simulink model "pumaModel"  (R2021b)
settings: Solver=VariableStepAuto  StartTime=0.0  StopTime=stopTime  FixedStep=.0001  RelTol=1e-3
values from neighbouring files (symbols this model uses):
  C = [0 c12_1*dq1 c13_1*dq3;c11_2*dq1 0 c22_2*dq2+c23_2*dq3;c11_3*dq1 c22_3*dq2 0]    [puma560ModifiedDynamics.m]
  dq_0 = [0 0 0]    [matlab.mat]
  fdControl = 2    [InitializationScript.m]
  fEE = 0    [InitializationScript.m]    (also in matlab.mat = 100)
  IC = [0;0;0]    [InitializationScript.m]    (also in matlab.mat = [0 0 0])
  m = 3    [matlab.mat]
  pathPoints = [IC,solution1,solution2,solution3,solution4,solution5,solution6]    [InitializationScript.m]    (also in matlab.mat = [0 0 0 4.71238898038 -1.57079632679 3.14159265359 3.14159265)
  q_0 = [0 0 0]    [matlab.mat]
  timePoints = [0 2 4 6 8 10 12]    [InitializationScript.m]    (also in matlab.mat = [0 2 4 6 8])
  velPoints = zeros(3,7)    [InitializationScript.m]    (also in matlab.mat = [0 0 0 0 0 0 0 0 0 0 0 0 ... (15 elements, 3x5)])
  X = [cos(q1)*(l2*cos(q2)+l3*sin(q2+q3));sin(q1)*(l2*cos(q2)+l3*sin(q2+q3));l1-l2*sin(q2)+l3*cos(q2+q3)]    [puma560ModifiedDynamics.m]
  Y = sym(zeros(3,size(cat(2,Y1,Y2,Y3),2)))    [puma560ModifiedDynamics.m]
undefined symbols (not defined in the file or in its folder): Z
libraries: sm_lib x96, nesl_utility x60, simulink x7, robotmaniplib x1, robotcorelib x1
(part 1 of 5)
PostSaveFcn:
  | save VariantSettings.mat
settings Model: VariantConfigurationObject=PUMA560VariantSettings  Creator=Chris  LastModifiedBy=Chris
settings SolverCC: AlgebraicLoopSolver=LineSearch
settings DebuggingCC: SFMachineParentedDataDiag=warning

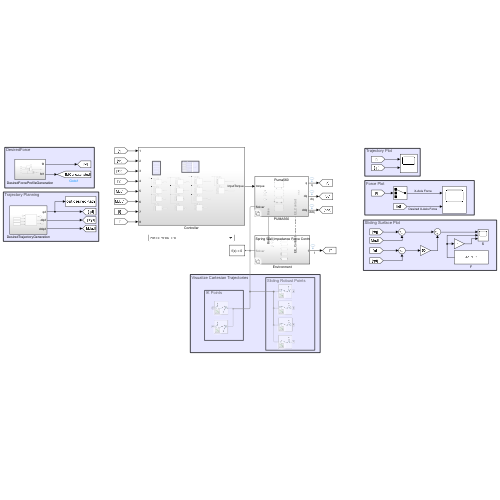
[thumbnail: Simulink's stored preview of the top-level diagram]
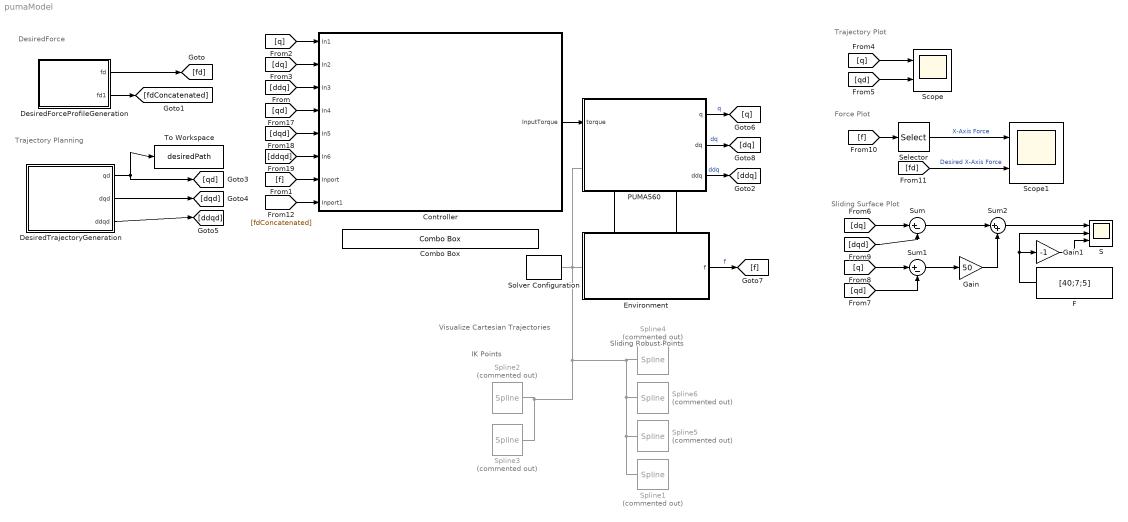
== system pumaModel ==
  note: Visualize Cartesian Trajectories
  note: DesiredForce
  note: Sliding Surface Plot
  note: Trajectory Plot
  note: Sliding Robust Points
  note: IK Points
  note: Trajectory Planning
  note: Force Plot
  Combo Box : ComboBox  LabelPosition=Hide  SelectedLabel=Parrellel Motion Force
      settings: Values={{'Inverse Torque', 'Lyapunov Torque', 'Impedance Joint Space', 'Impedance Task Space', 'Adaptive Control', 'PD + Gravity', 'Impedance Task State', 'Robust Control', 'Parrellel Motion Force', 'Task Space Impedance With Measurements', 'Sliding Robust Controller', 'Hybrid Force Motion', 'Hybrid Impedance Motion Control', 'Hybrid Impedance Force Control'}, [1 2 3 4 5 6 7 8 9 10 11 12 13 14]}
  Controller : Subsystem
  DesiredForceProfileGeneration : Subsystem
  DesiredTrajectoryGeneration : Subsystem
  Environment : Subsystem  Variant=on
      settings: PortSchema="{\"entries\":[{\"content\":{\"sides\":[{\"content\":{\"connectorIds\":[\"LConn1\"]},\"type\":\"ConnectorPlacement.EquallySpacedRectSide\",\"uuid\":\"bb63e962-d15f-4f0f-af2b-d9166a575433\"},{\"content\":{\"connectorIds\":[\"Out1\"],\"side\":\"RIGHT\"},\"type\":\"ConnectorPlacement.EquallySpacedRectSide\",\"uuid\":\"5f217ea6-af7d-4c7c-9fae-005e6a80c75a\"},{\"content\":{\"connectorIds\":[\"LConn2\",\"LConn3\"],\"side\":\"TOP\"},\"type\":\"ConnectorPlacement.EquallySpacedRectSide\",\"uuid\":\"72e5d329-ee37-4049-b27a-f006421b2cb1\"},{\"content\":{\"connectorIds\":[],\"side\":\"HIDDEN\"},\"type\":\"ConnectorPlacement.EquallySpacedRectSide\",\"uuid\":\"fb212f45-e29a-441e-a219-fbabe0f84998\"}]},\"type\":\"ConnectorPlacement.EquallySpacedConnector\",\"uuid\":\"6d8f9ed1-4648-49c1-a401-abad2abde741\"}],\"packageUris\":[\"http://schema.mathworks.com/mf0/Connector/R2020b\"],\"version\":\"1.0\"}"
  F : Constant  Value=[40;7;5]
  Gain : Gain  Gain=50
  Gain1 : Gain  Gain=-1
  PUMA560 : Subsystem  Variant=on
      settings: PortSchema="{\"entries\":[{\"content\":{\"sides\":[{\"content\":{\"connectorIds\":[\"In1\",\"LConn1\"]},\"type\":\"ConnectorPlacement.EquallySpacedRectSide\",\"uuid\":\"c7b40478-8afa-4d90-abdc-2a1179e0c85a\"},{\"content\":{\"connectorIds\":[\"Out1\",\"Out2\",\"Out3\"],\"side\":\"RIGHT\"},\"type\":\"ConnectorPlacement.EquallySpacedRectSide\",\"uuid\":\"fe05b273-9859-45af-b8f0-bcdecff42ea9\"},{\"content\":{\"connectorIds\":[],\"side\":\"TOP\"},\"type\":\"ConnectorPlacement.EquallySpacedRectSide\",\"uuid\":\"8295939b-ed6c-494a-8f2d-0843651cca51\"},{\"content\":{\"connectorIds\":[\"RConn1\",\"RConn2\"],\"side\":\"BOTTOM\"},\"type\":\"ConnectorPlacement.EquallySpacedRectSide\",\"uuid\":\"fbe51ea0-cfb2-4db3-ab8e-748ba1c11ce6\"},{\"content\":{\"connectorIds\":[],\"side\":\"HIDDEN\"},\"type\":\"ConnectorPlacement.EquallySpacedRectSide\",\"uuid\":\"fa6272a3-c07c-42c1-8bc0-64c7f45ab8c0\"}]},\"type\":\"ConnectorPlacement.EquallySpacedConnector\",\"uuid\":\"730599d1-a108-4fea-aae7-88428ae8f259\"}],\"packageUris\":[\"http://schema.mathworks.com/mf0/Connector/R2020b\"],\"version\":\"1.0\"}"
  S : Scope  NumInputPorts=3
  Scope : Scope  NumInputPorts=2
  Scope1 : Scope  NumInputPorts=2
  Selector : Selector  InputPortWidth=3  IndexOptions=Index vector (dialog)  Indices=[1]  OutputSizes=1
  Solver Configuration : nesl_utility/Solver Configuration  PhysicalDomain=network_engine_domain  SubClassName=solver  LeftPortType=input  RightPortType=generic  Tones=[]  Harmonics=[]  SimulateNoise=off  Profile=off  UseLocalSampling=off  EnableSwitchedLinearOptims=on  FrequencyDomain=off  UseCCode=off  RelTol=0.001  AbsTol=1e-06  MinStep=1e-09  ToWorkspace=off  RevertToSquareIcSolve=off  NumHomotopyIterations=100  PhasorMode=off  PhasorModeNumHarmonics=1  DoDC=off  ResidualTolerance=1e-09  UseLocalSolver=off  LocalSolverChoice=NE_PARTITIONING_ADVANCER  LocalSolverSampleTime=0.001  DoFixedCost=off  MaxNonlinIter=3  MaxModeIter=2  ComputeImpulses=off  ImpulseIterations=2  LinearAlgebra=auto  EquationFormulation=NE_TIME_EF  DelaysMemoryBudget=1024  AutomaticFiltering=on  FilteringTimeConstant=0.001  PartitionStorageMethod=AS_NEEDED  PartitionMemoryBudget=1024  PartitionMethod=ROBUST
      settings: SourceProductBaseCode=PW,SS
  Spline1 : sm_lib/Curves and Surfaces/Spline  Commented=on  GraphicAmbientColor=[0.15 0.15 0.15 1.0]  GraphicDiffuseColor=[1.0 1.0 0.0]  DataPoints=out.xTrajectory.Data  DataPointsUnits=m  GraphicEmissiveColor=[0.0 0.0 0.0 1.0]  EndConditionType=Natural  MarkerShape=Sphere  MarkerSize=10  GraphicType=FromGeometry  GraphicOpacity=1.0  GraphicShininess=75  GraphicSpecularColor=[0.5 0.5 0.5 1.0]  GraphicVisPropType=SimpleVisualProperties
  Spline2 : sm_lib/Curves and Surfaces/Spline  Commented=on  GraphicAmbientColor=[0.15 0.15 0.15 1.0]  GraphicDiffuseColor=[0.2 1.0 0.0]  DataPoints=preSetPointsDesired  DataPointsUnits=m  GraphicEmissiveColor=[0.0 0.0 0.0 1.0]  EndConditionType=Natural  MarkerShape=Sphere  MarkerSize=10  GraphicType=FromGeometry  GraphicOpacity=1.0  GraphicShininess=75  GraphicSpecularColor=[0.5 0.5 0.5 1.0]  GraphicVisPropType=SimpleVisualProperties
  Spline3 : sm_lib/Curves and Surfaces/Spline  Commented=on  GraphicAmbientColor=[0.15 0.15 0.15 1.0]  GraphicDiffuseColor=[1.0 0.0 0.2]  DataPoints=preSetPointsIK  DataPointsUnits=m  GraphicEmissiveColor=[0.0 0.0 0.0 1.0]  EndConditionType=Natural  MarkerShape=Sphere  MarkerSize=10  GraphicType=FromGeometry  GraphicOpacity=1.0  GraphicShininess=75  GraphicSpecularColor=[0.5 0.5 0.5 1.0]  GraphicVisPropType=SimpleVisualProperties
  Spline4 : sm_lib/Curves and Surfaces/Spline  Commented=on  GraphicAmbientColor=[0.15 0.15 0.15 1.0]  GraphicDiffuseColor=[1.0 0.0 0.2]  DataPoints=robustControlPoints_IK  DataPointsUnits=m  GraphicEmissiveColor=[0.0 0.0 0.0 1.0]  EndConditionType=Natural  MarkerShape=Sphere  MarkerSize=10  GraphicType=FromGeometry  GraphicOpacity=1.0  GraphicShininess=75  GraphicSpecularColor=[0.5 0.5 0.5 1.0]  GraphicVisPropType=SimpleVisualProperties
  Spline5 : sm_lib/Curves and Surfaces/Spline  Commented=on  GraphicAmbientColor=[0.15 0.15 0.15 1.0]  GraphicDiffuseColor=[0.0 1.0 0.2]  DataPoints=fEEPoints  DataPointsUnits=m  GraphicEmissiveColor=[0.0 0.0 0.0 1.0]  EndConditionType=Natural  MarkerShape=Sphere  MarkerSize=10  GraphicType=FromGeometry  GraphicOpacity=1.0  GraphicShininess=75  GraphicSpecularColor=[0.5 0.5 0.5 1.0]  GraphicVisPropType=SimpleVisualProperties
  Spline6 : sm_lib/Curves and Surfaces/Spline  Commented=on  GraphicAmbientColor=[0.15 0.15 0.15 1.0]  GraphicDiffuseColor=[1.0 1.0 0.0]  DataPoints=robustControlPoints  DataPointsUnits=m  GraphicEmissiveColor=[0.0 0.0 0.0 1.0]  EndConditionType=Natural  MarkerShape=Sphere  MarkerSize=10  GraphicType=FromGeometry  GraphicOpacity=1.0  GraphicShininess=75  GraphicSpecularColor=[0.5 0.5 0.5 1.0]  GraphicVisPropType=SimpleVisualProperties
  Sum : Sum  Inputs=|+-
  Sum1 : Sum  Inputs=|+-
  Sum2 : Sum  Inputs=|++
  To Workspace : ToWorkspace  VariableName=desiredPath  SaveFormat=Timeseries  SampleTime=.1
  wires:
  [dqd] -> Controller/5(In5)
  [ddqd] -> Controller/6(In6)
  [q] -> Controller/1(In1)
  [dq] -> Controller/2(In2)
  [qd] -> Controller/4(In4)
  [ddq] -> Controller/3(In3)
  [f] -> Controller/7(Inport)
  Controller/1(InputTorque) -> PUMA560/1(torque)
  PUMA560/2(dq) -> [dq]  "dq"
  PUMA560/3(ddq) -> [ddq]  "ddq"
  PUMA560/1(q) -> [q]  "q"
  Environment/1(f) -> [f]  "f"
  [q] -> Scope/1
  [qd] -> Scope/2
  [dq] -> Sum/1
  [q] -> Sum1/1
  [dqd] -> Sum/2
  [qd] -> Sum1/2
  Sum1/1 -> Gain/1
  Sum/1 -> Sum2/1
  Gain/1 -> Sum2/2
  Sum2/1 -> S/1
  [fd] -> Scope1/2  "Desired X-Axis Force"
  Selector/1 -> Scope1/1  "X-Axis Force"
  F/1 -> S/2, Gain1/1
  Gain1/1 -> S/3
  [f] -> Selector/1
  [fdConcatenated] -> Controller/8(Inport1)
  DesiredForceProfileGeneration/1(fd) -> [fd]
  DesiredForceProfileGeneration/2(fd1) -> [fdConcatenated]
  DesiredTrajectoryGeneration/1(qd) -> To Workspace/1, [qd]
  DesiredTrajectoryGeneration/2(dqd) -> [dqd]
  DesiredTrajectoryGeneration/3(ddqd) -> [ddqd]
  connections:
  Environment/LConn2 -- PUMA560/RConn1
  Environment/LConn3 -- PUMA560/RConn2
  Spline5/LConn1 -- Spline1/LConn1 -- Spline6/LConn1 -- Spline3/LConn1 -- Spline2/LConn1 -- Solver Configuration/RConn1 -- PUMA560/LConn1 -- Environment/LConn1 -- Spline4/LConn1

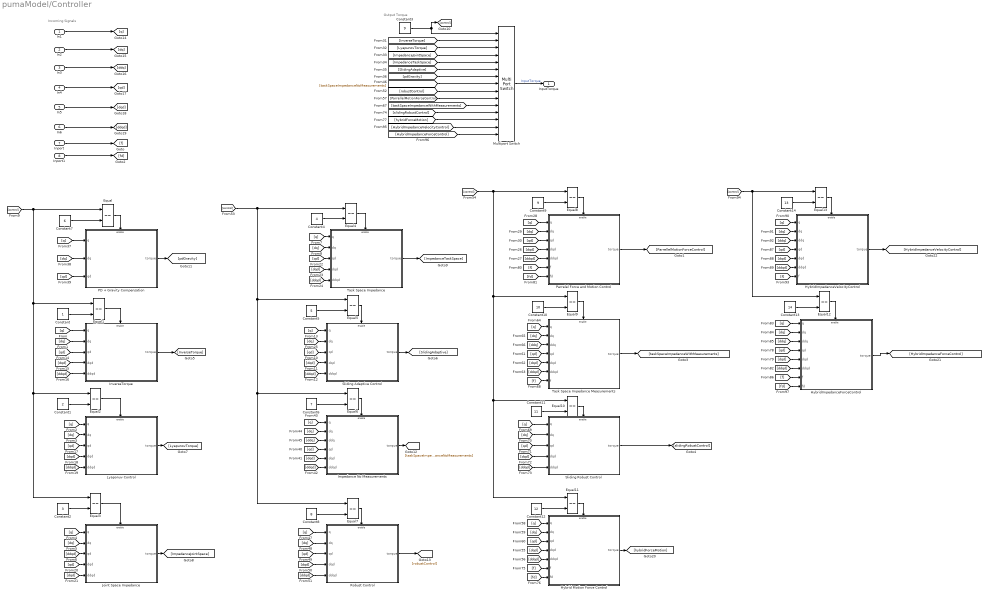
== system pumaModel/Controller ==
  note: Output Torque
  note: Incoming Signals
  In1 : Inport
  In2 : Inport  Port=2
  In3 : Inport  Port=3
  In4 : Inport  Port=4
  In5 : Inport  Port=5
  In6 : Inport  Port=6
  Inport : Inport  Port=7
  Inport1 : Inport  Port=8
  Constant : Constant
  Constant1 : Constant  Value=2
  Constant10 : Constant  Value=10
  Constant11 : Constant  Value=11
  Constant12 : Constant  Value=12
  Constant13 : Constant  Value=14
  Constant14 : Constant  Value=13
  Constant2 : Constant  Value=3
  Constant3 : Constant  Value=9
  Constant4 : Constant  Value=4
  Constant5 : Constant  Value=5
  Constant6 : Constant  Value=7
  Constant7 : Constant  Value=6
  Constant8 : Constant  Value=8
  Constant9 : Constant  Value=9
  Equal{,1..13} (14 alike) : RelationalOperator  Operator===  OutDataTypeStr=boolean  RndMeth=Simplest
  Hybrid Motion Force Control : Subsystem
  HybridImpedanceForceControl : Subsystem
  HybridImpedanceVelocityControl : Subsystem
  Impedance No Measurements : Subsystem
  InverseTorque : Subsystem
  Joint Space Impedance : Subsystem
  Lyaponuv Control : Subsystem
  Multiport Switch : MultiPortSwitch  Inputs=14
  PD + Gravity Compensation : Subsystem
  Parrelel Force and Motion Control : Subsystem
  Robust Control : Subsystem
  Sliding Adaptive Control : Subsystem
  Sliding Robust Control : Subsystem
  Task Space Impedance : Subsystem
  Task Space Impedance Measurements : Subsystem
  InputTorque : Outport
  wires:
  [dqd] -> Joint Space Impedance/5(ddqd)
  Constant3/1 -> [control], Multiport Switch/1
  [q] -> Robust Control/1(q)
  [qd] -> InverseTorque/3(qd)
  [dqd] -> Impedance No Measurements/5(dqd)
  [dq] -> Task Space Impedance/2(dq)
  [dqd] -> InverseTorque/4(dqd)
  [ddqd] -> Joint Space Impedance/3(qd)
  [ddqd] -> Impedance No Measurements/6(ddqd)
  Lyaponuv Control/1(torque) -> [LyapunovTorque]
  [q] -> Joint Space Impedance/1(q)
  [InverseTorque] -> Multiport Switch/2
  [dqd] -> Lyaponuv Control/4(dqd)
  [q] -> InverseTorque/1(q)
  [LyapunovTorque] -> Multiport Switch/3
  [qd] -> Lyaponuv Control/3(qd)
  [dq] -> Joint Space Impedance/2(dq)
  Joint Space Impedance/1(torque) -> [ImpedanceJointSpace]
  [ImpedanceJointSpace] -> Multiport Switch/4
  [q] -> Lyaponuv Control/1(q)
  [dq] -> InverseTorque/2(dq)
  [qd] -> Joint Space Impedance/4(dqd)
  [ddqd] -> Task Space Impedance/5(ddqd)
  [SlidingAdaptive] -> Multiport Switch/6
  [dqd] -> Robust Control/4(dqd)
  [qd] -> Impedance No Measurements/4(qd)
  [ImpedanceTaskSpace] -> Multiport Switch/5
  [robustControl] -> Multiport Switch/9
  [q] -> Impedance No Measurements/1(q)
  [dq] -> Lyaponuv Control/2(dq)
  [pdGravity] -> Multiport Switch/7
  Task Space Impedance/1(torque) -> [ImpedanceTaskSpace]
  Robust Control/1(torque) -> [robustControl]
  [ddqd] -> InverseTorque/5(ddqd)
  [ddqd] -> Robust Control/5(ddqd)
  [qd] -> Task Space Impedance/3(qd)
  [q] -> Task Space Impedance/1(q)
  [dq] -> Robust Control/2(dq)
  [ddq] -> Impedance No Measurements/3(ddq)
  [dq] -> Impedance No Measurements/2(dq)
  [qd] -> Robust Control/3(qd)
  [dqd] -> Task Space Impedance/4(dqd)
  [ddqd] -> Lyaponuv Control/5(ddqd)
  [taskSpaceImpedanceNoMeasurements] -> Multiport Switch/8
  In2/1 -> [dq]
  In3/1 -> [ddq]
  In4/1 -> [qd]
  In5/1 -> [dqd]
  In6/1 -> [ddqd]
  In1/1 -> [q]
  Multiport Switch/1 -> InputTorque/1  "InputTorque"
  Inport/1 -> [f]
  [ParrellelMotionForceControl] -> Multiport Switch/10
  Inport1/1 -> [fd]
  [dq] -> Task Space Impedance Measurements/2(dq)
  [ddq] -> Task Space Impedance Measurements/3(ddq)
  Task Space Impedance Measurements/1(torque) -> [taskSpaceImpedanceWithMeasurements]
  [q] -> Task Space Impedance Measurements/1(q)
  [qd] -> Task Space Impedance Measurements/4(qd)
  [ddqd] -> Task Space Impedance Measurements/6(ddqd)
  [dqd] -> Task Space Impedance Measurements/5(dqd)
  [taskSpaceImpedanceWithMeasurements] -> Multiport Switch/11
  [f] -> Task Space Impedance Measurements/7(f)
  [qd] -> Sliding Robust Control/3(qd)
  [dq] -> Sliding Robust Control/2(dq)
  [ddqd] -> Sliding Robust Control/5(ddqd)
  Sliding Robust Control/1(torque) -> [slidingRobustControl]
  [dqd] -> Sliding Robust Control/4(dqd)
  [q] -> Sliding Robust Control/1(q)
  [q] -> PD + Gravity Compensation/1(q)
  [dq] -> PD + Gravity Compensation/2(dq)
  [qd] -> PD + Gravity Compensation/3(qd)
  PD + Gravity Compensation/1(torque) -> [pdGravity]
  InverseTorque/1(torque) -> [InverseTorque]
  Sliding Adaptive Control/1(torque) -> [SlidingAdaptive]
  [q] -> Sliding Adaptive Control/1(q)
  [dq] -> Sliding Adaptive Control/2(dq)
  [dqd] -> Sliding Adaptive Control/4(dqd)
  [ddqd] -> Sliding Adaptive Control/5(ddqd)
  Impedance No Measurements/1(torque) -> [taskSpaceImpedanceNoMeasurements]
  [q] -> Parrelel Force and Motion Control/1(q)
  [dq] -> Parrelel Force and Motion Control/2(dq)
  [qd] -> Parrelel Force and Motion Control/3(qd)
  [dqd] -> Parrelel Force and Motion Control/4(dqd)
  [ddqd] -> Parrelel Force and Motion Control/5(ddqd)
  [f] -> Parrelel Force and Motion Control/6(f)
  [fd] -> Parrelel Force and Motion Control/7(fd)
  Parrelel Force and Motion Control/1(torque) -> [ParrellelMotionForceControl]
  Equal/1 -> PD + Gravity Compensation/Enable
  Equal1/1 -> InverseTorque/Enable
  Constant/1 -> Equal1/2
  Equal2/1 -> Lyaponuv Control/Enable
  Constant1/1 -> Equal2/2
  Constant2/1 -> Equal3/2
  Equal3/1 -> Joint Space Impedance/Enable
  Equal4/1 -> Task Space Impedance/Enable
  Constant4/1 -> Equal4/2
  Equal5/1 -> Sliding Adaptive Control/Enable
  Constant5/1 -> Equal5/2
  Constant6/1 -> Equal6/2
  Equal6/1 -> Impedance No Measurements/Enable
  [control] -> Equal3/1, Equal2/1, Equal1/1, Equal/1
  Constant7/1 -> Equal/2
  [control] -> Equal7/1, Equal6/1, Equal5/1, Equal4/1
  Equal7/1 -> Robust Control/Enable
  Constant8/1 -> Equal7/2
  Constant9/1 -> Equal8/2
  Equal8/1 -> Parrelel Force and Motion Control/Enable
  Equal9/1 -> Task Space Impedance Measurements/Enable
  Constant10/1 -> Equal9/2
  Constant11/1 -> Equal10/2
  Equal10/1 -> Sliding Robust Control/Enable
  [qd] -> Sliding Adaptive Control/3(qd)
  [slidingRobustControl] -> Multiport Switch/12
  [q] -> Hybrid Motion Force Control/1(q)
  [dq] -> Hybrid Motion Force Control/2(dq)
  [qd] -> Hybrid Motion Force Control/3(qd)
  [dqd] -> Hybrid Motion Force Control/4(dqd)
  [ddqd] -> Hybrid Motion Force Control/5(ddqd)
  [f] -> Hybrid Motion Force Control/6(f)
  [fd] -> Hybrid Motion Force Control/7(fd)
  Equal11/1 -> Hybrid Motion Force Control/Enable
  Constant12/1 -> Equal11/2
  [control] -> Equal11/1, Equal10/1, Equal9/1, Equal8/1
  [hybridForceMotion] -> Multiport Switch/13
  Hybrid Motion Force Control/1(torque) -> [hybridForceMotion]
  Constant13/1 -> Equal12/2
  Equal12/1 -> HybridImpedanceForceControl/Enable
  [f] -> HybridImpedanceForceControl/7(f)
  [dqd] -> HybridImpedanceForceControl/5(dqd)
  [ddqd] -> HybridImpedanceForceControl/6(ddqd)
  [qd] -> HybridImpedanceForceControl/4(qd)
  [q] -> HybridImpedanceForceControl/1(q)
  HybridImpedanceForceControl/1(torque) -> [HybridImpedanceForceControl]
  [ddq] -> HybridImpedanceForceControl/3(ddq)
  [dq] -> HybridImpedanceForceControl/2(dq)
  [dq] -> HybridImpedanceVelocityControl/2(dq)
  [ddq] -> HybridImpedanceVelocityControl/3(ddq)
  HybridImpedanceVelocityControl/1(torque) -> [HybridImpedanceVelocityControl]
  [q] -> HybridImpedanceVelocityControl/1(q)
  [qd] -> HybridImpedanceVelocityControl/4(qd)
  [ddqd] -> HybridImpedanceVelocityControl/6(ddqd)
  [dqd] -> HybridImpedanceVelocityControl/5(dqd)
  [f] -> HybridImpedanceVelocityControl/7(f)
  Equal13/1 -> HybridImpedanceVelocityControl/Enable
  Constant14/1 -> Equal13/2
  [control] -> Equal12/1, Equal13/1
  [HybridImpedanceForceControl] -> Multiport Switch/15
  [HybridImpedanceVelocityControl] -> Multiport Switch/14
  [fd] -> HybridImpedanceForceControl/8(fd)

== system pumaModel/DesiredForceProfileGeneration ==
  Force Trajectory Control : Constant  Value=fdControl
  ForceImpdeanceForces : simulink/Sources/Repeating Sequence Stair  OutValues=[0 25 25 35 35 0 0 0].'  tsamp=2  OutMin=[]  OutMax=[]  OutDataTypeStr=double  OutputDataTypeScalingMode=double  OutDataType=fixdt(0,8)  ConRadixGroup=Best Precision: Vector-wise  OutScaling=2^-12
  HybridForces : simulink/Sources/Repeating Sequence Stair  OutValues=[0 20 20 20 30 30 30 20 20].'  tsamp=2  OutMin=[]  OutMax=[]  OutDataTypeStr=double  OutputDataTypeScalingMode=double  OutDataType=fixdt(0,8)  ConRadixGroup=Best Precision: Vector-wise  OutScaling=2^-12
  Multiport Switch : MultiPortSwitch
  Vector Concatenate : Concatenate  NumInputs=3
  Zero : Constant  Value=0  OutDataTypeStr=Inherit: Inherit via back propagation
  fd : Outport
  fd1 : Outport  Port=2
  wires:
  Zero/1 -> Multiport Switch/4, Vector Concatenate/3, Vector Concatenate/2
  HybridForces/1 -> Multiport Switch/3
  Multiport Switch/1 -> fd/1, Vector Concatenate/1  "fd"
  ForceImpdeanceForces/1 -> Multiport Switch/2
  Vector Concatenate/1 -> fd1/1  "fd"
  Force Trajectory Control/1 -> Multiport Switch/1

== system pumaModel/DesiredTrajectoryGeneration ==
  Clock : Clock
  Constant1 : Constant  Value=timePoints
  Constant2 : Constant  Value=velPoints
  From IK Solver : Constant  Value=pathPoints
  Polynomial Trajectory : robotcorelib/Polynomial Trajectory  WaypointSource=External  Waypoints=zeros(3,5)  TimePoints=[0,2,4,6,8]  TimeInterval=[ 1, 4 ]  Method=Cubic Polynomial  ParameterSource=External  VelocityBoundaryCondition=zeros(3, 7)  AccelerationBoundaryCondition=zeros( 3,7 )  SimulateUsing=Interpreted execution
  qd : Outport
  dqd : Outport  Port=2
  ddqd : Outport  Port=3
  wires:
  Polynomial Trajectory/2 -> dqd/1  "dqd"
  From IK Solver/1 -> Polynomial Trajectory/2
  Clock/1 -> Polynomial Trajectory/1
  Polynomial Trajectory/1 -> qd/1  "qd"
  Constant1/1 -> Polynomial Trajectory/3
  Constant2/1 -> Polynomial Trajectory/4
  Polynomial Trajectory/3 -> ddqd/1  "ddqd"

== system pumaModel/Environment ==
  EmptyEnvironment : Subsystem  VariantControl=EmptyEnvironment
  Moving Wall (Impedance Demo) : Subsystem  VariantControl=MovingWallXDirection
  SinusoidalMovingWall : Subsystem  VariantControl=SinusoidalMovingWallXDirection
  Spring Wall (Robust Demo) : Subsystem  VariantControl=SpringWallRobustDemo
  Spring Wall Impedance Force Control : Subsystem  VariantControl=ImpedanceForceDemo
  Solver : PMIOPort  Tag=PMCPort  Side=Left
  Base : PMIOPort  Tag=PMCPort  Port=2  Side=Left
  EE_Contact : PMIOPort  Tag=PMCPort  Port=3  Side=Left
  f : Outport

== system pumaModel/PUMA560 ==
  torque : Inport
  Manipulator Dynamic : Subsystem  VariantControl=Puma560Model
      settings: PortSchema="{\"entries\":[{\"content\":{\"sides\":[{\"content\":{\"connectorIds\":[\"In1\",\"LConn1\"]},\"type\":\"ConnectorPlacement.EquallySpacedRectSide\",\"uuid\":\"c7b40478-8afa-4d90-abdc-2a1179e0c85a\"},{\"content\":{\"connectorIds\":[\"Out1\",\"Out2\",\"Out3\"],\"side\":\"RIGHT\"},\"type\":\"ConnectorPlacement.EquallySpacedRectSide\",\"uuid\":\"fe05b273-9859-45af-b8f0-bcdecff42ea9\"},{\"content\":{\"connectorIds\":[],\"side\":\"TOP\"},\"type\":\"ConnectorPlacement.EquallySpacedRectSide\",\"uuid\":\"8295939b-ed6c-494a-8f2d-0843651cca51\"},{\"content\":{\"connectorIds\":[\"RConn1\",\"RConn2\"],\"side\":\"BOTTOM\"},\"type\":\"ConnectorPlacement.EquallySpacedRectSide\",\"uuid\":\"8036e508-5d94-4d22-863a-5395a38bd792\"},{\"content\":{\"connectorIds\":[],\"side\":\"HIDDEN\"},\"type\":\"ConnectorPlacement.EquallySpacedRectSide\",\"uuid\":\"fa6272a3-c07c-42c1-8bc0-64c7f45ab8c0\"}]},\"type\":\"ConnectorPlacement.EquallySpacedConnector\",\"uuid\":\"730599d1-a108-4fea-aae7-88428ae8f259\"}],\"packageUris\":[\"http://schema.mathworks.com/mf0/Connector/R2020b\"],\"version\":\"1.0\"}"
  Puma560 : Subsystem  VariantControl=Puma560Robot
      settings: PortSchema="{\"entries\":[{\"content\":{\"sides\":[{\"content\":{\"connectorIds\":[\"In1\",\"LConn1\"]},\"type\":\"ConnectorPlacement.EquallySpacedRectSide\",\"uuid\":\"eeb4ec5f-56a2-4f26-ab6d-42dca043b0dc\"},{\"content\":{\"connectorIds\":[\"Out1\",\"Out2\",\"Out3\"],\"side\":\"RIGHT\"},\"type\":\"ConnectorPlacement.EquallySpacedRectSide\",\"uuid\":\"a05aa011-ba43-4273-a182-008499cb643c\"},{\"content\":{\"connectorIds\":[],\"side\":\"TOP\"},\"type\":\"ConnectorPlacement.EquallySpacedRectSide\",\"uuid\":\"feb1388d-d90f-4c23-b0d1-a9b953ab65a0\"},{\"content\":{\"connectorIds\":[\"RConn1\",\"RConn2\"],\"side\":\"BOTTOM\"},\"type\":\"ConnectorPlacement.EquallySpacedRectSide\",\"uuid\":\"b97d61d2-16b2-4c0e-9bea-7da5346b0e14\"},{\"content\":{\"connectorIds\":[],\"side\":\"HIDDEN\"},\"type\":\"ConnectorPlacement.EquallySpacedRectSide\",\"uuid\":\"f19c9757-bb55-405d-82cd-459dd882f530\"}]},\"type\":\"ConnectorPlacement.EquallySpacedConnector\",\"uuid\":\"e536172a-20b5-41b8-b384-221a917f8e88\"}],\"packageUris\":[\"http://schema.mathworks.com/mf0/Connector/R2020b\"],\"version\":\"1.0\"}"
  Puma560PlannerCOM : Subsystem  VariantControl=Puma560Planner
      settings: PortSchema="{\"entries\":[{\"content\":{\"sides\":[{\"content\":{\"connectorIds\":[\"In1\",\"LConn1\"]},\"type\":\"ConnectorPlacement.EquallySpacedRectSide\",\"uuid\":\"eeb4ec5f-56a2-4f26-ab6d-42dca043b0dc\"},{\"content\":{\"connectorIds\":[\"Out1\",\"Out2\",\"Out3\"],\"side\":\"RIGHT\"},\"type\":\"ConnectorPlacement.EquallySpacedRectSide\",\"uuid\":\"a05aa011-ba43-4273-a182-008499cb643c\"},{\"content\":{\"connectorIds\":[],\"side\":\"TOP\"},\"type\":\"ConnectorPlacement.EquallySpacedRectSide\",\"uuid\":\"feb1388d-d90f-4c23-b0d1-a9b953ab65a0\"},{\"content\":{\"connectorIds\":[\"RConn1\",\"RConn2\"],\"side\":\"BOTTOM\"},\"type\":\"ConnectorPlacement.EquallySpacedRectSide\",\"uuid\":\"b97d61d2-16b2-4c0e-9bea-7da5346b0e14\"},{\"content\":{\"connectorIds\":[],\"side\":\"HIDDEN\"},\"type\":\"ConnectorPlacement.EquallySpacedRectSide\",\"uuid\":\"f19c9757-bb55-405d-82cd-459dd882f530\"}]},\"type\":\"ConnectorPlacement.EquallySpacedConnector\",\"uuid\":\"e536172a-20b5-41b8-b384-221a917f8e88\"}],\"packageUris\":[\"http://schema.mathworks.com/mf0/Connector/R2020b\"],\"version\":\"1.0\"}"
  Simplified Puma : Subsystem  VariantControl=Puma560Simplified
  Base : PMIOPort  Tag=PMCPort  Side=Right
  EE_Contact : PMIOPort  Tag=PMCPort  Port=2  Side=Right
  Solver : PMIOPort  Tag=PMCPort  Port=3  Side=Left
  q : Outport
  dq : Outport  Port=2
  ddq : Outport  Port=3

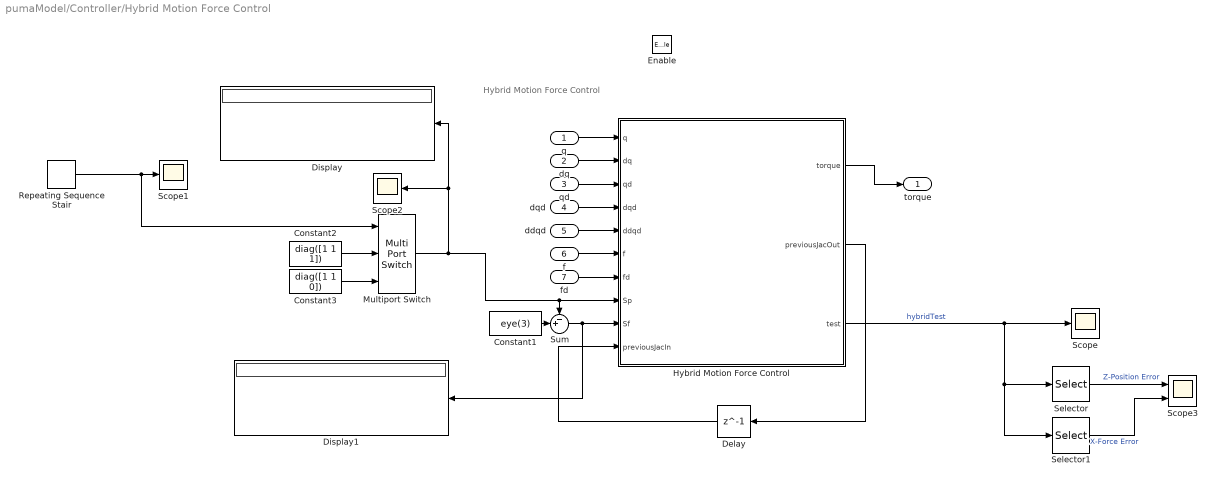
== system pumaModel/Controller/Hybrid Motion Force Control ==
  note: Hybrid Motion Force Control
  q : Inport
  dq : Inport  Port=2
  qd : Inport  Port=3
  dqd : Inport  Port=4
  ddqd : Inport  Port=5
  f : Inport  Port=6
  fd : Inport  Port=7
  Enable : EnablePort
  Constant1 : Constant  Value=eye(3)
  Constant2 : Constant  Value=diag([1 1 1])
  Constant3 : Constant  Value=diag([1 1 0])
  Delay : Delay  DelayLength=1  InitialCondition=zeros(3)
  Display : Display
  Display1 : Display
  Hybrid Motion Force Control : MATLAB Function  TreatAsAtomicUnit=on
  Multiport Switch : MultiPortSwitch  Inputs=2
  Repeating Sequence Stair : simulink/Sources/Repeating Sequence Stair  OutValues=[1 2 2 2 2 2 2].'  tsamp=2  OutMin=[]  OutMax=[]  OutDataTypeStr=double  OutputDataTypeScalingMode=double  OutDataType=fixdt(0,8)  ConRadixGroup=Best Precision: Vector-wise  OutScaling=2^-12
  Scope : Scope
  Scope1 : Scope
  Scope2 : Scope
  Scope3 : Scope  NumInputPorts=2
  Selector : Selector  NumberOfDimensions=2  InputPortWidth=[3,2]  IndexOptions=Index vector (dialog),Index vector (dialog)  Indices=[3],1  OutputSizes=1,1
  Selector1 : Selector  NumberOfDimensions=2  InputPortWidth=[3,2]  IndexOptions=Index vector (dialog),Index vector (dialog)  Indices=[1],2  OutputSizes=1,1
  Sum : Sum  Inputs=-+|
  torque : Outport
  wires:
  Delay/1 -> Hybrid Motion Force Control/10(previousJacIn)
  Hybrid Motion Force Control/2(previousJacOut) -> Delay/1
  Hybrid Motion Force Control/1(torque) -> torque/1
  ddqd/1 -> Hybrid Motion Force Control/5(ddqd)
  dqd/1 -> Hybrid Motion Force Control/4(dqd)
  qd/1 -> Hybrid Motion Force Control/3(qd)
  dq/1 -> Hybrid Motion Force Control/2(dq)
  q/1 -> Hybrid Motion Force Control/1(q)
  f/1 -> Hybrid Motion Force Control/6(f)
  fd/1 -> Hybrid Motion Force Control/7(fd)
  Constant1/1 -> Sum/2
  Constant3/1 -> Multiport Switch/3
  Repeating Sequence Stair/1 -> Multiport Switch/1, Scope1/1
  Sum/1 -> Display1/1, Hybrid Motion Force Control/9(Sf)
  Multiport Switch/1 -> Scope2/1, Display/1, Hybrid Motion Force Control/8(Sp), Sum/1
  Constant2/1 -> Multiport Switch/2
  Hybrid Motion Force Control/3(test) -> Selector1/1, Selector/1, Scope/1  "hybridTest"
  Selector/1 -> Scope3/1  "Z-Position Error"
  Selector1/1 -> Scope3/2  "X-Force Error"

== system pumaModel/Controller/HybridImpedanceForceControl ==
  q : Inport
  dq : Inport  Port=2
  ddq : Inport  Port=3
  qd : Inport  Port=4
  dqd : Inport  Port=5
  ddqd : Inport  Port=6
  f : Inport  Port=7
  fd : Inport  Port=8
  Enable : EnablePort
  Hybrid Impedance Force Control : MATLAB Function  TreatAsAtomicUnit=on
  torque : Outport
  wires:
  f/1 -> Hybrid Impedance Force Control/7(f)
  ddqd/1 -> Hybrid Impedance Force Control/6(ddqd)
  dqd/1 -> Hybrid Impedance Force Control/5(dqd)
  qd/1 -> Hybrid Impedance Force Control/4(qd)
  dq/1 -> Hybrid Impedance Force Control/2(dq)
  q/1 -> Hybrid Impedance Force Control/1(q)
  Hybrid Impedance Force Control/1(torque) -> torque/1
  ddq/1 -> Hybrid Impedance Force Control/3(ddq)
  fd/1 -> Hybrid Impedance Force Control/8(fd)

== system pumaModel/Controller/HybridImpedanceVelocityControl ==
  q : Inport
  dq : Inport  Port=2
  ddq : Inport  Port=3
  qd : Inport  Port=4
  dqd : Inport  Port=5
  ddqd : Inport  Port=6
  f : Inport  Port=7
  Enable : EnablePort
  Hybrid Impedance Velocity Control : MATLAB Function  TreatAsAtomicUnit=on
  torque : Outport
  wires:
  ddq/1 -> Hybrid Impedance Velocity Control/3(ddq)
  Hybrid Impedance Velocity Control/1(torque) -> torque/1
  q/1 -> Hybrid Impedance Velocity Control/1(q)
  dq/1 -> Hybrid Impedance Velocity Control/2(dq)
  qd/1 -> Hybrid Impedance Velocity Control/4(qd)
  dqd/1 -> Hybrid Impedance Velocity Control/5(dqd)
  ddqd/1 -> Hybrid Impedance Velocity Control/6(ddqd)
  f/1 -> Hybrid Impedance Velocity Control/7(f)

== system pumaModel/Controller/Impedance No Measurements ==
  q : Inport
  dq : Inport  Port=2
  ddq : Inport  Port=3
  qd : Inport  Port=4
  dqd : Inport  Port=5
  ddqd : Inport  Port=6
  Enable : EnablePort
  Scope : Scope
  TaskSpaceImpedance_NoMeasurements : MATLAB Function  TreatAsAtomicUnit=on
  Unit Delay : UnitDelay  InitialCondition=ones(3)  SampleTime=-1  HasFrameUpgradeWarning=on
  torque : Outport
  wires:
  dqd/1 -> TaskSpaceImpedance_NoMeasurements/5(dqd)
  ddqd/1 -> TaskSpaceImpedance_NoMeasurements/6(ddqd)
  dq/1 -> TaskSpaceImpedance_NoMeasurements/2(dq)
  qd/1 -> TaskSpaceImpedance_NoMeasurements/4(qd)
  TaskSpaceImpedance_NoMeasurements/1(torque) -> torque/1
  q/1 -> TaskSpaceImpedance_NoMeasurements/1(q)
  TaskSpaceImpedance_NoMeasurements/2(previousJacOut) -> Unit Delay/1
  Unit Delay/1 -> TaskSpaceImpedance_NoMeasurements/7(previousJacIn)
  ddq/1 -> TaskSpaceImpedance_NoMeasurements/3(ddq)
  TaskSpaceImpedance_NoMeasurements/3(Hp) -> Scope/1

== system pumaModel/Controller/InverseTorque ==
  q : Inport
  dq : Inport  Port=2
  qd : Inport  Port=3
  dqd : Inport  Port=4
  ddqd : Inport  Port=5
  Enable : EnablePort
  InverseTorque : MATLAB Function  TreatAsAtomicUnit=on
  torque : Outport
  wires:
  dqd/1 -> InverseTorque/4(dqd)
  ddqd/1 -> InverseTorque/5(ddqd)
  dq/1 -> InverseTorque/2(dq)
  qd/1 -> InverseTorque/3(qd)
  InverseTorque/1(torque) -> torque/1
  q/1 -> InverseTorque/1(q)

== system pumaModel/Controller/Joint Space Impedance ==
  q : Inport
  dq : Inport  Port=2
  qd : Inport  Port=3
  dqd : Inport  Port=4
  ddqd : Inport  Port=5
  Enable : EnablePort
  ImpedanceControllerJointSpace : MATLAB Function  TreatAsAtomicUnit=on
  torque : Outport
  wires:
  dqd/1 -> ImpedanceControllerJointSpace/4(qd)
  ddqd/1 -> ImpedanceControllerJointSpace/5(dqd)
  dq/1 -> ImpedanceControllerJointSpace/2(dq)
  qd/1 -> ImpedanceControllerJointSpace/3(ddqd)
  ImpedanceControllerJointSpace/1(torque) -> torque/1
  q/1 -> ImpedanceControllerJointSpace/1(q)

== system pumaModel/Controller/Lyaponuv Control ==
  q : Inport
  dq : Inport  Port=2
  qd : Inport  Port=3
  dqd : Inport  Port=4
  ddqd : Inport  Port=5
  Enable : EnablePort
  Lyapanov : MATLAB Function  TreatAsAtomicUnit=on
  torque : Outport
  wires:
  dqd/1 -> Lyapanov/4(dqd)
  ddqd/1 -> Lyapanov/5(ddqd)
  dq/1 -> Lyapanov/2(dq)
  qd/1 -> Lyapanov/3(qd)
  Lyapanov/1(torque) -> torque/1
  q/1 -> Lyapanov/1(q)

== system pumaModel/Controller/PD + Gravity Compensation ==
  q : Inport
  dq : Inport  Port=2
  qd : Inport  Port=3
  Enable : EnablePort
  PD + Gravity Compensation : Subsystem
      settings: PortSchema="{\"entries\":[{\"content\":{\"sides\":[{\"content\":{\"connectorIds\":[\"In1\"]},\"type\":\"ConnectorPlacement.EquallySpacedRectSide\",\"uuid\":\"76ddbea7-8326-45c4-b454-c13a7194c229\"},{\"content\":{\"connectorIds\":[\"Out1\"],\"side\":\"RIGHT\"},\"type\":\"ConnectorPlacement.EquallySpacedRectSide\",\"uuid\":\"f5586d01-1ac4-444a-a8ff-727324082b97\"},{\"content\":{\"connectorIds\":[\"In2\",\"In3\"],\"side\":\"TOP\"},\"type\":\"ConnectorPlacement.EquallySpacedRectSide\",\"uuid\":\"14cfcb35-c5a5-4a3c-8697-71e5c86b6ab2\"},{\"content\":{\"connectorIds\":[],\"side\":\"HIDDEN\"},\"type\":\"ConnectorPlacement.EquallySpacedRectSide\",\"uuid\":\"b757ed73-e1fc-4cf1-9ad4-f48cba7d72ed\"}]},\"type\":\"ConnectorPlacement.EquallySpacedConnector\",\"uuid\":\"f2c76c78-31f9-4c22-a4be-0d563828d323\"}],\"packageUris\":[\"http://schema.mathworks.com/mf0/Connector/R2020b\"],\"version\":\"1.0\"}"
  torque : Outport
  wires:
  dq/1 -> PD + Gravity Compensation/2(dq)
  qd/1 -> PD + Gravity Compensation/1(qd)
  PD + Gravity Compensation/1(torque) -> torque/1
  q/1 -> PD + Gravity Compensation/3(q)

== system pumaModel/Controller/Parrelel Force and Motion Control ==
  note: Parrellel Force & Motion Control
  q : Inport
  dq : Inport  Port=2
  qd : Inport  Port=3
  dqd : Inport  Port=4
  ddqd : Inport  Port=5
  f : Inport  Port=6
  fd : Inport  Port=7
  Enable : EnablePort
  Delay : Delay  DelayLength=1  InitialCondition=zeros(3)
  Force Control : Subsystem
  Parrellel Decompostion+Tracking Control+ID : MATLAB Function  TreatAsAtomicUnit=on
  Scope : Scope  NumInputPorts=3
  Scope1 : Scope
  torque : Outport
  wires:
  f/1 -> Parrellel Decompostion+Tracking Control+ID/9(f), Force Control/1(F)
  q/1 -> Parrellel Decompostion+Tracking Control+ID/1(q)
  dq/1 -> Parrellel Decompostion+Tracking Control+ID/2(dq)
  qd/1 -> Parrellel Decompostion+Tracking Control+ID/3(qd)
  dqd/1 -> Parrellel Decompostion+Tracking Control+ID/4(dqd)
  ddqd/1 -> Parrellel Decompostion+Tracking Control+ID/5(ddqd)
  fd/1 -> Force Control/2(Fd)
  Force Control/3(pfDotDot) -> Parrellel Decompostion+Tracking Control+ID/8(ddpf), Scope/3
  Parrellel Decompostion+Tracking Control+ID/1(torque) -> torque/1
  Parrellel Decompostion+Tracking Control+ID/2(previousJacOut) -> Delay/1
  Force Control/1(pf) -> Parrellel Decompostion+Tracking Control+ID/6(pf), Scope/1
  Force Control/2(pfDot) -> Parrellel Decompostion+Tracking Control+ID/7(dpf), Scope/2
  Delay/1 -> Parrellel Decompostion+Tracking Control+ID/10(previousJacIn)
  Parrellel Decompostion+Tracking Control+ID/3(test) -> Scope1/1

== system pumaModel/Controller/Robust Control ==
  q : Inport
  dq : Inport  Port=2
  qd : Inport  Port=3
  dqd : Inport  Port=4
  ddqd : Inport  Port=5
  Enable : EnablePort
  RobustControl : MATLAB Function  TreatAsAtomicUnit=on
  torque : Outport
  wires:
  q/1 -> RobustControl/1(q)
  RobustControl/1(u) -> torque/1
  qd/1 -> RobustControl/3(qd)
  dq/1 -> RobustControl/2(dq)
  ddqd/1 -> RobustControl/5(ddqd)
  dqd/1 -> RobustControl/4(dqd)

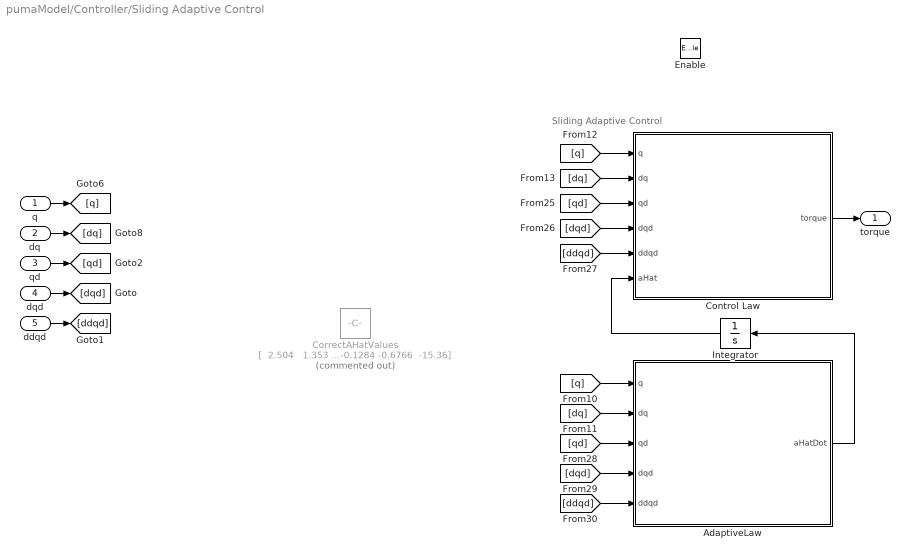
== system pumaModel/Controller/Sliding Adaptive Control ==
  note: Sliding Adaptive Control
  q : Inport
  dq : Inport  Port=2
  qd : Inport  Port=3
  dqd : Inport  Port=4
  ddqd : Inport  Port=5
  Enable : EnablePort
  AdaptiveLaw : MATLAB Function  TreatAsAtomicUnit=on
  Control Law : MATLAB Function  TreatAsAtomicUnit=on
  CorrectAHatValues : Constant  Commented=on  Value=|
      | [  2.504
      |   1.353
      |  0.2569
      |   0.302
      |  0.2569
      |   1.353
      |    -1.0
      |  -2.504
      |   1.353
      |  0.2569
      |   1.353
      |    2.76
      |  0.6766
      |  0.2569
      | -0.1284
      |  -1.353
      |   2.504
      |   1.353
      |  0.6766
      |  -73.23
      |  -15.36
      |  0.6766
      |  0.2569
      |  0.2569
      | -0.3383
      | -0.1284
      | -0.6766
      |  -15.36]
  Integrator : Integrator
  torque : Outport
  wires:
  dqd/1 -> [dqd]
  ddqd/1 -> [ddqd]
  dq/1 -> [dq]
  Control Law/1(torque) -> torque/1
  q/1 -> [q]
  [ddqd] -> AdaptiveLaw/5(ddqd)
  [dq] -> AdaptiveLaw/2(dq)
  [dqd] -> Control Law/4(dqd)
  [ddqd] -> Control Law/5(ddqd)
  [dqd] -> AdaptiveLaw/4(dqd)
  [qd] -> Control Law/3(qd)
  Integrator/1 -> Control Law/6(aHat)
  [qd] -> AdaptiveLaw/3(qd)
  AdaptiveLaw/1(aHatDot) -> Integrator/1
  [q] -> AdaptiveLaw/1(q)
  [dq] -> Control Law/2(dq)
  [q] -> Control Law/1(q)
  qd/1 -> [qd]

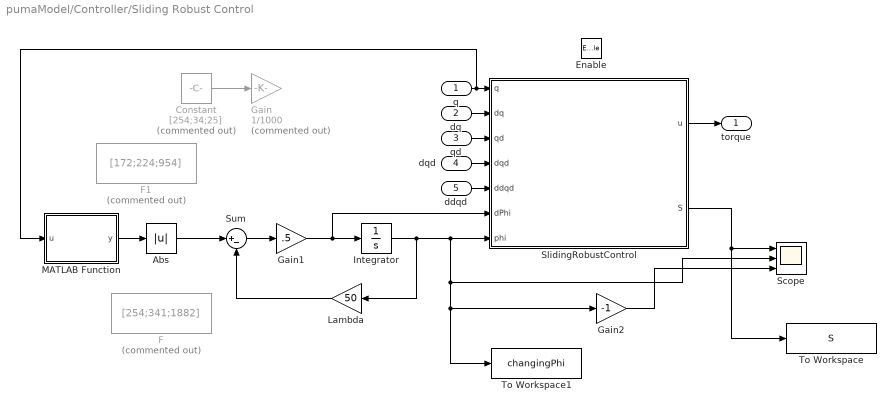
== system pumaModel/Controller/Sliding Robust Control ==
  q : Inport
  dq : Inport  Port=2
  qd : Inport  Port=3
  dqd : Inport  Port=4
  ddqd : Inport  Port=5
  Enable : EnablePort
  Abs : Abs
  Constant : Constant  Commented=on  Value=[254;34;25]
  F : Constant  Commented=on  Value=[254;341;1882]
  F1 : Constant  Commented=on  Value=[172;224;954]
  Gain : Gain  Commented=on  Gain=1/1000
  Gain1 : Gain  Gain=.5
  Gain2 : Gain  Gain=-1
  Integrator : Integrator  InitialCondition=[1;1;1]
  Lambda : Gain  Gain=50
  MATLAB Function : MATLAB Function  TreatAsAtomicUnit=on
  Scope : Scope  NumInputPorts=3
  SlidingRobustControl : MATLAB Function  TreatAsAtomicUnit=on
  Sum : Sum  Inputs=|+-
  To Workspace : ToWorkspace  VariableName=S  SaveFormat=Timeseries  SampleTime=-1
  To Workspace1 : ToWorkspace  VariableName=changingPhi  SaveFormat=Timeseries  SampleTime=-1
  torque : Outport
  wires:
  dqd/1 -> SlidingRobustControl/4(dqd)
  ddqd/1 -> SlidingRobustControl/5(ddqd)
  dq/1 -> SlidingRobustControl/2(dq)
  qd/1 -> SlidingRobustControl/3(qd)
  q/1 -> MATLAB Function/1(u), SlidingRobustControl/1(q)
  Integrator/1 -> Scope/2, To Workspace1/1, Gain2/1, SlidingRobustControl/7(phi), Lambda/1
  Lambda/1 -> Sum/2
  Constant/1 -> Gain/1
  Sum/1 -> Gain1/1
  Gain1/1 -> SlidingRobustControl/6(dPhi), Integrator/1
  SlidingRobustControl/1(u) -> torque/1
  SlidingRobustControl/2(S) -> To Workspace/1, Scope/1
  MATLAB Function/1(y) -> Abs/1
  Gain2/1 -> Scope/3
  Abs/1 -> Sum/1

== system pumaModel/Controller/Task Space Impedance ==
  q : Inport
  dq : Inport  Port=2
  qd : Inport  Port=3
  dqd : Inport  Port=4
  ddqd : Inport  Port=5
  Enable : EnablePort
  ImpedanceControllerTaskSpace : MATLAB Function  TreatAsAtomicUnit=on
  torque : Outport
  wires:
  dqd/1 -> ImpedanceControllerTaskSpace/4(dqd)
  ddqd/1 -> ImpedanceControllerTaskSpace/5(ddqd)
  dq/1 -> ImpedanceControllerTaskSpace/2(dq)
  qd/1 -> ImpedanceControllerTaskSpace/3(qd)
  ImpedanceControllerTaskSpace/1(torque) -> torque/1
  q/1 -> ImpedanceControllerTaskSpace/1(q)

== system pumaModel/Controller/Task Space Impedance Measurements ==
  q : Inport
  dq : Inport  Port=2
  ddq : Inport  Port=3
  qd : Inport  Port=4
  dqd : Inport  Port=5
  ddqd : Inport  Port=6
  f : Inport  Port=7
  Enable : EnablePort
  TaskSpaceImpedance_withMeasurements : MATLAB Function  TreatAsAtomicUnit=on
  torque : Outport
  wires:
  ddq/1 -> TaskSpaceImpedance_withMeasurements/3(ddq)
  TaskSpaceImpedance_withMeasurements/1(torque) -> torque/1
  q/1 -> TaskSpaceImpedance_withMeasurements/1(q)
  dq/1 -> TaskSpaceImpedance_withMeasurements/2(dq)
  qd/1 -> TaskSpaceImpedance_withMeasurements/4(qd)
  dqd/1 -> TaskSpaceImpedance_withMeasurements/5(dqd)
  ddqd/1 -> TaskSpaceImpedance_withMeasurements/6(ddqd)
  f/1 -> TaskSpaceImpedance_withMeasurements/7(f)

== system pumaModel/Environment/EmptyEnvironment ==
  Base : PMIOPort  Side=Left
  EE_Contact : PMIOPort  Port=2  Side=Left

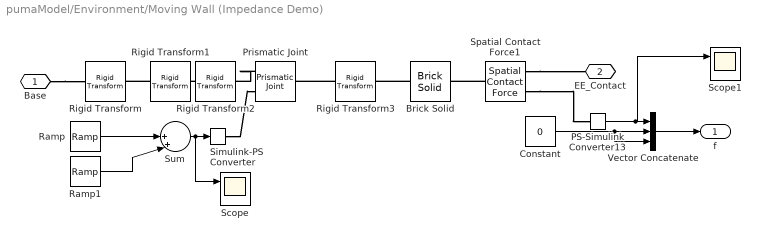
== system pumaModel/Environment/Moving Wall (Impedance Demo) ==
  Brick Solid : sm_lib/Body Elements/Brick Solid  GraphicAmbientColor=[0.15 0.15 0.15 1.0]  BasedOnType=Density  BrickDimensions=[0.05,1.5,1.5]  BrickDimensionUnits=m  CenterOfMass=[0 0 0]  CenterOfMassUnits=m  GraphicDiffuseColor=[0.4 1.0 1.0]  Density=1000  DensityUnits=kg/m^3  DoExposeReferenceFrame=on  GraphicEmissiveColor=[0.0 0.0 0.0 1.0]  ExportEntireGeometry=on  SerializedFrames=<Frames/>  MarkerShape=Sphere  MarkerSize=10  GraphicType=FromGeometry  InertiaType=PointMass  Mass=1  MassUnits=kg  MomentsOfInertia=[1 1 1]  MomentsOfInertiaUnits=kg*m^2  GraphicOpacity=1.0  ProductsOfInertia=[0 0 0]  ProductsOfInertiaUnits=kg*m^2  GraphicShininess=75  GraphicSpecularColor=[0.5 0.5 0.5 1.0]  GraphicVisPropType=SimpleVisualProperties
  Constant : Constant  Value=0
  PS-Simulink Converter13 : nesl_utility/PS-Simulink Converter  PhysicalDomain=network_engine_domain  SubClassName=ps_output  LeftPortType=input  RightPortType=output  PseudoPeriodic=off  Frequencies=[]  Unit=inherit  AffineConversion=off
      settings: SourceProductBaseCode=PW,SS
  Prismatic Joint : sm_lib/Joints/Prismatic Joint  JointMode=Normal  SenseConstraintForce=off  SenseConstraintForceX=off  SenseConstraintForceY=off  SenseConstraintForceZ=off  SenseConstraintTorque=off  SenseConstraintTorqueX=off  SenseConstraintTorqueY=off  SenseConstraintTorqueZ=off  SenseTotalForce=off  SenseTotalForceX=off  SenseTotalForceY=off  SenseTotalForceZ=off  SenseTotalTorque=off  SenseTotalTorqueX=off  SenseTotalTorqueY=off  SenseTotalTorqueZ=off  CompositeWrenchDir=FollowerOnBase  CompositeWrenchFrame=BaseFrame  EquilibriumPosition=0  EquilibriumPositionUnits=m  SpringStiffness=0  SpringStiffnessUnits=N/m  DampingCoefficient=0  DampingCoefficientUnits=N/(m/s)  TorqueActuationMode=InputTorque  MotionActuationMode=ComputedMotion  SensePosition=off  SenseVelocity=off  SenseAcceleration=off  SenseTorqueForce=off  SenseLowerLimitTorqueForce=off  SenseUpperLimitTorqueForce=off  LowerLimitSpecify=off  LowerLimitBound=-1  LowerLimitBoundUnits=m  LowerLimitStiffness=1e6  LowerLimitStiffnessUnits=N/m  LowerLimitDamping=1e3  LowerLimitDampingUnits=N/(m/s)  LowerLimitTransitionRegionWidth=1e-4  LowerLimitTransitionRegionWidthUnits=m  UpperLimitSpecify=off  UpperLimitBound=1  UpperLimitBoundUnits=m  UpperLimitStiffness=1e6  UpperLimitStiffnessUnits=N/m  UpperLimitDamping=1e3  UpperLimitDampingUnits=N/(m/s)  UpperLimitTransitionRegionWidth=1e-4  UpperLimitTransitionRegionWidthUnits=m  PositionTargetSpecify=off  PositionTargetPriority=High  PositionTargetValue=0  PositionTargetValueUnits=m  VelocityTargetSpecify=off  VelocityTargetPriority=High  VelocityTargetValue=0  VelocityTargetValueUnits=m/s
  Ramp : simulink/Sources/Ramp  slope=-5  start=2  InitialOutput=0
  Ramp1 : simulink/Sources/Ramp  slope=5  start=6  InitialOutput=0
  Rigid Transform : sm_lib/Frames and Transforms/Rigid Transform  TranslationMethod=StandardAxis  TranslationStandardOffset=.75  TranslationLengthUnit=m  TranslationStandardAxis=+Z  TranslationCartesianOffset=[0 0 0]  TranslationROffset=0  TranslationROffsetUnits=m  TranslationZOffset=0  TranslationZOffsetUnits=m  TranslationThetaOffset=0  TranslationThetaOffsetUnits=deg  RotationMethod=None  RotationAngleUnits=deg  RotationStandardAxis=+Z  RotationAngle=0.0  RotationArbitraryAxis=[0 0 1]  FollAlignAxisA=+X  BaseAlignAxisA=+Y  FollAlignAxisB=+Y  BaseAlignAxisB=+Z  RotationSequenceAxes=FollowerAxes  RotationSequence=XYX  RotationSequenceAngles=[0 0 0]  RotationSequenceAnglesUnits=deg  RotationMatrix=[1 0 0; 0 1 0; 0 0 1]
  Rigid Transform1 : sm_lib/Frames and Transforms/Rigid Transform  TranslationMethod=StandardAxis  TranslationStandardOffset=.75  TranslationLengthUnit=m  TranslationStandardAxis=+X  TranslationCartesianOffset=[0 0 0]  TranslationROffset=0  TranslationROffsetUnits=m  TranslationZOffset=0  TranslationZOffsetUnits=m  TranslationThetaOffset=0  TranslationThetaOffsetUnits=deg  RotationMethod=None  RotationAngleUnits=deg  RotationStandardAxis=+Z  RotationAngle=0.0  RotationArbitraryAxis=[0 0 1]  FollAlignAxisA=+X  BaseAlignAxisA=+Y  FollAlignAxisB=+Y  BaseAlignAxisB=+Z  RotationSequenceAxes=FollowerAxes  RotationSequence=XYX  RotationSequenceAngles=[0 0 0]  RotationSequenceAnglesUnits=deg  RotationMatrix=[1 0 0; 0 1 0; 0 0 1]
  Rigid Transform2 : sm_lib/Frames and Transforms/Rigid Transform  TranslationMethod=None  TranslationStandardOffset=.65  TranslationLengthUnit=m  TranslationStandardAxis=+X  TranslationCartesianOffset=[0 0 0]  TranslationROffset=0  TranslationROffsetUnits=m  TranslationZOffset=0  TranslationZOffsetUnits=m  TranslationThetaOffset=0  TranslationThetaOffsetUnits=deg  RotationMethod=StandardAxis  RotationAngleUnits=deg  RotationStandardAxis=+Y  RotationAngle=90  RotationArbitraryAxis=[0 0 1]  FollAlignAxisA=+X  BaseAlignAxisA=+Y  FollAlignAxisB=+Y  BaseAlignAxisB=+Z  RotationSequenceAxes=FollowerAxes  RotationSequence=XYX  RotationSequenceAngles=[0 0 0]  RotationSequenceAnglesUnits=deg  RotationMatrix=[1 0 0; 0 1 0; 0 0 1]
  Rigid Transform3 : sm_lib/Frames and Transforms/Rigid Transform  TranslationMethod=None  TranslationStandardOffset=.65  TranslationLengthUnit=m  TranslationStandardAxis=+X  TranslationCartesianOffset=[0 0 0]  TranslationROffset=0  TranslationROffsetUnits=m  TranslationZOffset=0  TranslationZOffsetUnits=m  TranslationThetaOffset=0  TranslationThetaOffsetUnits=deg  RotationMethod=StandardAxis  RotationAngleUnits=deg  RotationStandardAxis=+Y  RotationAngle=-90  RotationArbitraryAxis=[0 0 1]  FollAlignAxisA=+X  BaseAlignAxisA=+Y  FollAlignAxisB=+Y  BaseAlignAxisB=+Z  RotationSequenceAxes=FollowerAxes  RotationSequence=XYX  RotationSequenceAngles=[0 0 0]  RotationSequenceAnglesUnits=deg  RotationMatrix=[1 0 0; 0 1 0; 0 0 1]
  Scope : Scope  NumInputPorts=2
  Scope1 : Scope  NumInputPorts=2
  Simulink-PS Converter : nesl_utility/Simulink-PS Converter  PhysicalDomain=network_engine_domain  SubClassName=ps_input  LeftPortType=input  RightPortType=output  PseudoPeriodic=off  Frequencies=[]  NoiseDistribution=none  NoiseParameters=[]  Unit=1  AffineConversion=off  FilteringAndDerivatives=provide  SimscapeFilterOrder=1  InputFilterTimeConstant=0.001  UdotUserProvided=0
      settings: SourceProductBaseCode=PW,SS
  Spatial Contact Force1 : sm_lib/Forces and Torques/Spatial Contact Force  CoefficientOfDynamicFriction=0.3  CoefficientOfStaticFriction=0.5  SenseContactBaseRotation=off  SenseContactBaseTranslation=off  NormalDamping=1e3  NormalDampingUnits=N/(m/s)  SenseContactFollowerRotation=off  SenseContactFollowerTranslation=off  SenseContactSignal=off  NormalStiffness=1e6  NormalStiffnessUnits=N/m  FrictionalCriticalVelocity=1e-3  FrictionalCriticalVelocityUnits=m/s  ZeroCrossDetectContactStartAndEnd=off  FrictionType=SmoothStickSlip  SenseFrictionalForceMagnitude=off  SenseNormalForceMagnitude=on  NormalForceType=SmoothSpringDamper  SenseNormalVelocity=off  SenseSeparationDistance=off  SenseTangentialVelocity=off  SenseTangentialVelocityMagnitude=off  NormalTransitionRegionWidth=1e-4  NormalTransitionRegionWidthUnits=m
  Sum : Sum  Inputs=||++|
  Vector Concatenate : Concatenate  NumInputs=3
  Base : PMIOPort  Side=Left
  EE_Contact : PMIOPort  Port=2  Side=Left
  f : Outport
  wires:
  Ramp/1 -> Sum/1
  Sum/1 -> Scope/1, Simulink-PS Converter/1
  Ramp1/1 -> Sum/2
  PS-Simulink Converter13/1 -> Scope1/1, Vector Concatenate/1
  Constant/1 -> Vector Concatenate/2, Vector Concatenate/3
  Vector Concatenate/1 -> f/1
  connections:
  Base/RConn1 -- Rigid Transform/LConn1
  Rigid Transform2/LConn1 -- Rigid Transform1/RConn1
  Brick Solid/RConn1 -- Rigid Transform3/RConn1
  Prismatic Joint/LConn1 -- Rigid Transform2/RConn1
  Rigid Transform3/LConn1 -- Prismatic Joint/RConn1
  Rigid Transform1/LConn1 -- Rigid Transform/RConn1
  Simulink-PS Converter/RConn1 -- Prismatic Joint/LConn2
  Spatial Contact Force1/RConn1 -- EE_Contact/RConn1
  Spatial Contact Force1/RConn2 -- PS-Simulink Converter13/LConn1
  Spatial Contact Force1/LConn1 -- Brick Solid/LConn1
